simulink model "chap6_2sim"  (Simulink 8.1)
settings: Solver=ode45  StartTime=0.0  StopTime=10.0  RelTol=1e-3
settings Model: Creator=Administrator  LastModifiedBy=liujk
settings DataIOCC: SignalLoggingName=sigsOut
settings OptimizationCC: InitFltsAndDblsToZero=on
settings DebuggingCC: SaveWithParameterizedLinksMsg=none  SignalResolutionControl=TryResolveAllWithWarning  SolverPrmCheckMsg=none  MultiTaskDSMMsg=warning  MultiTaskCondExecSysMsg=none  StrictBusMsg=None
settings HardwareCC: TargetUnknown=on
settings RTWCC: IncludeERTFirstTime=on
settings GRTTargetCC: TargetFcnLib=ansi_tfl_tmw.mat

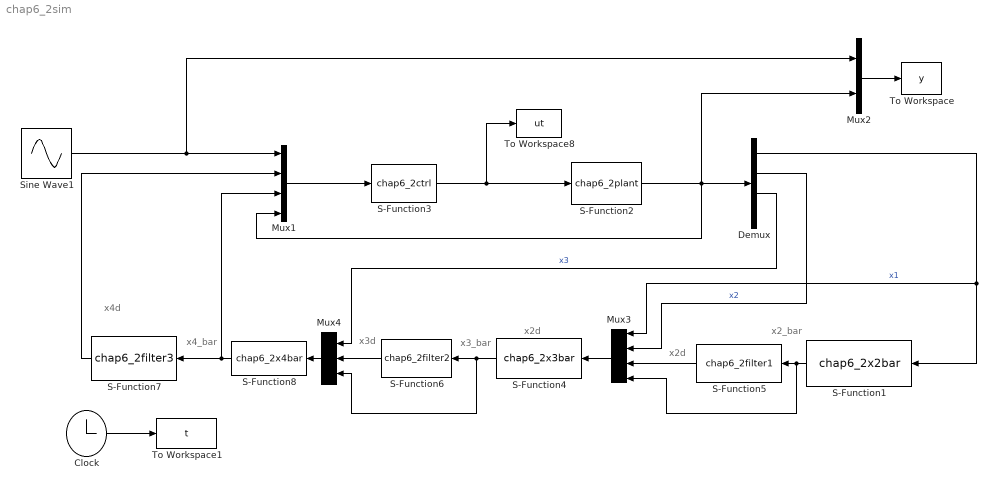
== system chap6_2sim ==
  note: x2d
  note: x2_bar
  note: x3_bar
  note: x3d
  note: x4_bar
  note: x4d
  note: x2d
  Clock : Clock
  Demux : Demux
  Mux1 : Mux
  Mux2 : Mux  Inputs=2
  Mux3 : Mux
  Mux4 : Mux  Inputs=3
  S-Function1 : S-Function  FunctionName=chap6_2x2bar  EnableBusSupport=off
  S-Function2 : S-Function  FunctionName=chap6_2plant  EnableBusSupport=off
  S-Function3 : S-Function  FunctionName=chap6_2ctrl  EnableBusSupport=off
  S-Function4 : S-Function  FunctionName=chap6_2x3bar  EnableBusSupport=off
  S-Function5 : S-Function  FunctionName=chap6_2filter1  EnableBusSupport=off
  S-Function6 : S-Function  FunctionName=chap6_2filter2  EnableBusSupport=off
  S-Function7 : S-Function  FunctionName=chap6_2filter3  EnableBusSupport=off
  S-Function8 : S-Function  FunctionName=chap6_2x4bar  EnableBusSupport=off
  Sine Wave1 : Sin  SampleTime=0
  To Workspace : ToWorkspace  VariableName=y  SampleTime=-1
  To Workspace1 : ToWorkspace  VariableName=t  SampleTime=-1
  To Workspace8 : ToWorkspace  VariableName=ut  SampleTime=-1
  wires:
  Clock/1 -> To Workspace1/1
  Mux1/1 -> S-Function3/1
  S-Function4/1 -> S-Function6/1, Mux4/3
  Sine Wave1/1 -> Mux1/1, Mux2/1
  S-Function2/1 -> Demux/1, Mux1/4, Mux2/2
  Demux/1 -> S-Function1/1, Mux3/1  "x1"
  Mux2/1 -> To Workspace/1
  S-Function3/1 -> S-Function2/1, To Workspace8/1
  Mux3/1 -> S-Function4/1
  Demux/3 -> Mux4/1  "x3"
  S-Function1/1 -> S-Function5/1, Mux3/4
  S-Function8/1 -> Mux1/3, S-Function7/1
  Mux4/1 -> S-Function8/1
  S-Function6/1 -> Mux4/2
  S-Function7/1 -> Mux1/2
  S-Function5/1 -> Mux3/3
  Demux/2 -> Mux3/2  "x2"
